simulink model "test_rig"  (Simulink 7.2)
settings: Solver=FixedStepDiscrete  StartTime=0.0  StopTime=55.0  FixedStep=0.5  RelTol=1e-3
libraries: simulink_need_slupdate x22, simulink x5, simulink_extras x1
settings Model: Creator=bjax  LastModifiedBy=bjax  ExtModeAutoUpdateStatusClock=off
settings DataIOCC: SignalLoggingName=sigsOut
settings OptimizationCC: InlineInvariantSignals=on  InitFltsAndDblsToZero=on
settings DebuggingCC: SaveWithParameterizedLinksMsg=none  SignalResolutionControl=TryResolveAllWithWarning  SolverPrmCheckMsg=none  MultiTaskDSMMsg=warning  MultiTaskCondExecSysMsg=none  StrictBusMsg=None
settings HardwareCC: TargetUnknown=on
settings RTWCC: IncludeERTFirstTime=on
settings GRTTargetCC: TargetFcnLib=ansi_tfl_tmw.mat  ModelReferenceCompliant=off  MatFileLogging=off

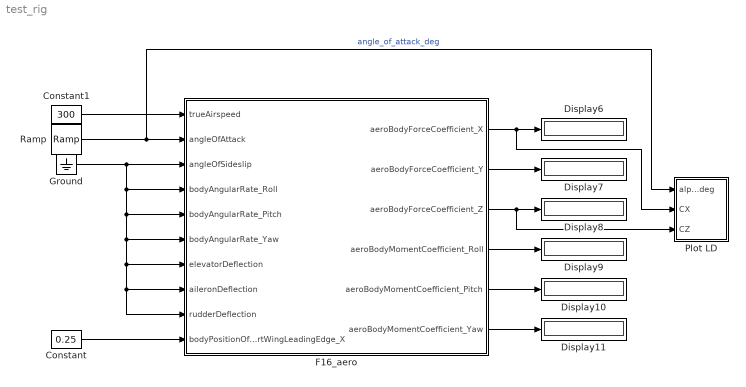
== system test_rig ==
  Constant : Constant  Value=0.25  OutDataType=sfix(16)  OutScaling=2^0
  Constant1 : Constant  Value=300  OutDataType=sfix(16)  OutScaling=2^0
  Display{6..11} (6 alike) : Display
  F16_aero : Subsystem
  Ground : Ground
  Plot LD : Subsystem
  Ramp : simulink/Sources/Ramp  SystemSampleTime=-1  slope=1  start=0  X0=-10
  wires:
  Ramp/1 -> Plot LD/1(alpha_deg), F16_aero/2(angleOfAttack)  "angle_of_attack_deg"
  F16_aero/2(aeroBodyForceCoefficient_Y) -> Display7/1
  F16_aero/3(aeroBodyForceCoefficient_Z) -> Display8/1, Plot LD/3(CZ)
  F16_aero/4(aeroBodyMomentCoefficient_Roll) -> Display9/1
  F16_aero/5(aeroBodyMomentCoefficient_Pitch) -> Display10/1
  F16_aero/6(aeroBodyMomentCoefficient_Yaw) -> Display11/1
  Constant/1 -> F16_aero/10(bodyPositionOfCgWrtWingLeadingEdge_X)
  Constant1/1 -> F16_aero/1(trueAirspeed)
  F16_aero/1(aeroBodyForceCoefficient_X) -> Display6/1, Plot LD/2(CX)
  Ground/1 -> F16_aero/8(aileronDeflection), F16_aero/9(rudderDeflection), F16_aero/7(elevatorDeflection), F16_aero/6(bodyAngularRate_Yaw), F16_aero/5(bodyAngularRate_Pitch), F16_aero/4(bodyAngularRate_Roll), F16_aero/3(angleOfSideslip)

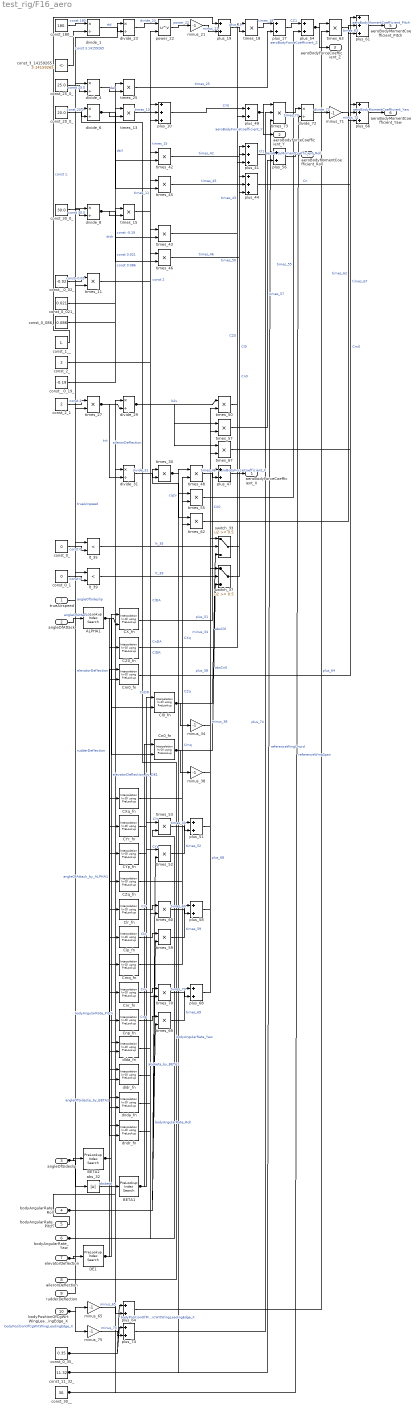
== system test_rig/F16_aero ==
  trueAirspeed : Inport
  angleOfAttack : Inport  Port=2
  angleOfSideslip : Inport  Port=3
  bodyAngularRate_Roll : Inport  Port=4
  bodyAngularRate_Pitch : Inport  Port=5
  bodyAngularRate_Yaw : Inport  Port=6
  elevatorDeflection : Inport  Port=7
  aileronDeflection : Inport  Port=8
  rudderDeflection : Inport  Port=9
  bodyPositionOfCgWrtWingLeadingEdge_X : Inport  Port=10
  ALPHA1 : simulink_need_slupdate/PreLookup Index Search  bpData=F16_aero_data.ALPHA1_pts  searchMode=Binary Search  cacheBpFlag=on  outputFlag=off  IndexDataType=uint32  extrapMode=Linear Extrapolation  rangeErrorMode=None
  BETA1 : simulink_need_slupdate/PreLookup Index Search  bpData=F16_aero_data.BETA1_pts  searchMode=Binary Search  cacheBpFlag=on  outputFlag=off  IndexDataType=uint32  extrapMode=Linear Extrapolation  rangeErrorMode=None
  BETA2 : simulink_need_slupdate/PreLookup Index Search  bpData=F16_aero_data.BETA2_pts  searchMode=Binary Search  cacheBpFlag=on  outputFlag=off  IndexDataType=uint32  extrapMode=Linear Extrapolation  rangeErrorMode=None
  CX_fn : simulink_need_slupdate/Interpolation (n-D) using PreLookup  numDimsPopupSelect=2  explicitNumDims=2  table=F16_aero_data.CX_table  interpMethod=Linear  extrapMethod=None - Clip  rangeErrorMode=None  NumSelectionDims=0
  CXq_fn : simulink_need_slupdate/Interpolation (n-D) using PreLookup  numDimsPopupSelect=1  explicitNumDims=1  table=F16_aero_data.CXq_table  interpMethod=Linear  extrapMethod=None - Clip  rangeErrorMode=None  NumSelectionDims=0
  CYp_fn : simulink_need_slupdate/Interpolation (n-D) using PreLookup  numDimsPopupSelect=1  explicitNumDims=1  table=F16_aero_data.CYp_table  interpMethod=Linear  extrapMethod=None - Clip  rangeErrorMode=None  NumSelectionDims=0
  CYr_fn : simulink_need_slupdate/Interpolation (n-D) using PreLookup  numDimsPopupSelect=1  explicitNumDims=1  table=F16_aero_data.CYr_table  interpMethod=Linear  extrapMethod=None - Clip  rangeErrorMode=None  NumSelectionDims=0
  CZ0_fn : simulink_need_slupdate/Interpolation (n-D) using PreLookup  numDimsPopupSelect=1  explicitNumDims=1  table=F16_aero_data.CZ0_table  interpMethod=Linear  extrapMethod=None - Clip  rangeErrorMode=None  NumSelectionDims=0
  CZq_fn : simulink_need_slupdate/Interpolation (n-D) using PreLookup  numDimsPopupSelect=1  explicitNumDims=1  table=F16_aero_data.CZq_table  interpMethod=Linear  extrapMethod=None - Clip  rangeErrorMode=None  NumSelectionDims=0
  Cl0_fn : simulink_need_slupdate/Interpolation (n-D) using PreLookup  numDimsPopupSelect=2  explicitNumDims=2  table=F16_aero_data.Cl0_table  interpMethod=Linear  extrapMethod=None - Clip  rangeErrorMode=None  NumSelectionDims=0
  Clp_fn : simulink_need_slupdate/Interpolation (n-D) using PreLookup  numDimsPopupSelect=1  explicitNumDims=1  table=F16_aero_data.Clp_table  interpMethod=Linear  extrapMethod=None - Clip  rangeErrorMode=None  NumSelectionDims=0
  Clr_fn : simulink_need_slupdate/Interpolation (n-D) using PreLookup  numDimsPopupSelect=1  explicitNumDims=1  table=F16_aero_data.Clr_table  interpMethod=Linear  extrapMethod=None - Clip  rangeErrorMode=None  NumSelectionDims=0
  Cm0_fn : simulink_need_slupdate/Interpolation (n-D) using PreLookup  numDimsPopupSelect=2  explicitNumDims=2  table=F16_aero_data.Cm0_table  interpMethod=Linear  extrapMethod=None - Clip  rangeErrorMode=None  NumSelectionDims=0
  Cmq_fn : simulink_need_slupdate/Interpolation (n-D) using PreLookup  numDimsPopupSelect=1  explicitNumDims=1  table=F16_aero_data.Cmq_table  interpMethod=Linear  extrapMethod=None - Clip  rangeErrorMode=None  NumSelectionDims=0
  Cn0_fn : simulink_need_slupdate/Interpolation (n-D) using PreLookup  numDimsPopupSelect=2  explicitNumDims=2  table=F16_aero_data.Cn0_table  interpMethod=Linear  extrapMethod=None - Clip  rangeErrorMode=None  NumSelectionDims=0
  Cnp_fn : simulink_need_slupdate/Interpolation (n-D) using PreLookup  numDimsPopupSelect=1  explicitNumDims=1  table=F16_aero_data.Cnp_table  interpMethod=Linear  extrapMethod=None - Clip  rangeErrorMode=None  NumSelectionDims=0
  Cnr_fn : simulink_need_slupdate/Interpolation (n-D) using PreLookup  numDimsPopupSelect=1  explicitNumDims=1  table=F16_aero_data.Cnr_table  interpMethod=Linear  extrapMethod=None - Clip  rangeErrorMode=None  NumSelectionDims=0
  DE1 : simulink_need_slupdate/PreLookup Index Search  bpData=F16_aero_data.DE1_pts  searchMode=Binary Search  cacheBpFlag=on  outputFlag=off  IndexDataType=uint32  extrapMode=Linear Extrapolation  rangeErrorMode=None
  abs_32 : Abs  SaturateOnIntegerOverflow=on
  const_0_ : Constant  Value=0
  const_0_021_ : Constant  Value=0.021
  const_0_086_ : Constant  Value=0.086
  const_0_1 : Constant  Value=0
  const_0_35_ : Constant  Value=0.35
  const_11_32_ : Constant  Value=11.32
  const_180__ : Constant  Value=180.
  const_1__ : Constant  Value=1.
  const_20_0_ : Constant  Value=20.0
  const_25_0_ : Constant  Value=25.0
  const_2_ : Constant  Value=2
  const_2_1 : Constant  Value=2
  const_30_0_ : Constant  Value=30.0
  const_30__ : Constant  Value=30.
  const_3_14159265_ : Constant  Value=3.14159265
  const__0_02_ : Constant  Value=-0.02
  const__0_19_ : Constant  Value=-0.19
  divide_{1,4,6,8,23,29,31,72} (8 alike) : Product  Inputs=*/  SaturateOnIntegerOverflow=on  RndMeth=Zero  InputSameDT=on  OutDataTypeStr=Inherit: Same as first input
  dlda_fn : simulink_need_slupdate/Interpolation (n-D) using PreLookup  numDimsPopupSelect=2  explicitNumDims=2  table=F16_aero_data.dlda_table  interpMethod=Linear  extrapMethod=None - Clip  rangeErrorMode=None  NumSelectionDims=0
  dldr_fn : simulink_need_slupdate/Interpolation (n-D) using PreLookup  numDimsPopupSelect=2  explicitNumDims=2  table=F16_aero_data.dldr_table  interpMethod=Linear  extrapMethod=None - Clip  rangeErrorMode=None  NumSelectionDims=0
  dnda_fn : simulink_need_slupdate/Interpolation (n-D) using PreLookup  numDimsPopupSelect=2  explicitNumDims=2  table=F16_aero_data.dnda_table  interpMethod=Linear  extrapMethod=None - Clip  rangeErrorMode=None  NumSelectionDims=0
  dndr_fn : simulink_need_slupdate/Interpolation (n-D) using PreLookup  numDimsPopupSelect=2  explicitNumDims=2  table=F16_aero_data.dndr_table  interpMethod=Linear  extrapMethod=None - Clip  rangeErrorMode=None  NumSelectionDims=0
  lt_35 : RelationalOperator  Operator=<  InputSameDT=on
  lt_39 : RelationalOperator  Operator=<  InputSameDT=on
  minus_{21,34,38,65,71,75} (6 alike) : Gain  Gain=-1  SaturateOnIntegerOverflow=on  OutDataTypeStr=Inherit: Same as input  ParamDataTypeStr=Inherit: Same as input
  plus_{10,41,44,61,66} (5 alike) : Sum  Inputs=+++  SaturateOnIntegerOverflow=on  InputSameDT=on  OutDataTypeStr=Inherit: Same as first input
  plus_{17,19,47,49,51,54,56,58,64,68,74} (11 alike) : Sum  SaturateOnIntegerOverflow=on  InputSameDT=on  OutDataTypeStr=Inherit: Same as first input
  power_22 : Math  Operator=pow  SaturateOnIntegerOverflow=on
  switch_33 : Switch  Threshold=0.5  SaturateOnIntegerOverflow=on  InputSameDT=on
  switch_37 : Switch  Threshold=0.5  SaturateOnIntegerOverflow=on  InputSameDT=on
  times_{11,13,15,18,25,27,30,42..43,45..46,48,50,52..53,55,57,59..60,62..63,67,69..70} (24 alike) : Product  SaturateOnIntegerOverflow=on  RndMeth=Zero  InputSameDT=on  OutDataTypeStr=Inherit: Same as first input
  times_73 : Product  Inputs=3  SaturateOnIntegerOverflow=on  RndMeth=Zero  InputSameDT=on  OutDataTypeStr=Inherit: Same as first input
  aeroBodyForceCoefficient_X : Outport
  aeroBodyForceCoefficient_Y : Outport  Port=2
  aeroBodyForceCoefficient_Z : Outport  Port=3
  aeroBodyMomentCoefficient_Roll : Outport  Port=4
  aeroBodyMomentCoefficient_Pitch : Outport  Port=5
  aeroBodyMomentCoefficient_Yaw : Outport  Port=6
  wires:
  BETA2/1 -> dndr_fn/1, dnda_fn/1, dldr_fn/1, dlda_fn/1  "angleOfSideslip_by_BETA2"
  BETA1/1 -> Cn0_fn/1, Cl0_fn/1  "absbeta_by_BETA1"
  ALPHA1/1 -> dndr_fn/2, dnda_fn/2, dldr_fn/2, dlda_fn/2, Cnp_fn/1, Cnr_fn/1, Cmq_fn/1, Clp_fn/1, Clr_fn/1, CZq_fn/1, CYp_fn/1, CYr_fn/1, CXq_fn/1, Cn0_fn/2, Cl0_fn/2, Cm0_fn/2, CZ0_fn/1, CX_fn/2  "angleOfAttack_by_ALPHA1"
  DE1/1 -> Cm0_fn/1, CX_fn/1  "elevatorDeflection_by_DE1"
  minus_75/1 -> plus_74/2  "minus_75"
  plus_74/1 -> times_73/2  "plus_74"
  times_73/1 -> divide_72/1  "times_73"
  divide_72/1 -> minus_71/1  "divide_72"
  minus_71/1 -> plus_66/3  "minus_71"
  times_70/1 -> plus_68/2  "times_70"
  times_69/1 -> plus_68/1  "times_69"
  plus_68/1 -> times_67/2  "plus_68"
  times_67/1 -> plus_66/2  "times_67"
  plus_66/1 -> aeroBodyMomentCoefficient_Yaw/1  "aeroBodyMomentCoefficient_Yaw"
  minus_65/1 -> plus_64/2  "minus_65"
  plus_64/1 -> times_63/2  "plus_64"
  times_63/1 -> plus_61/3  "times_63"
  times_62/1 -> plus_61/2  "times_62"
  plus_61/1 -> aeroBodyMomentCoefficient_Pitch/1  "aeroBodyMomentCoefficient_Pitch"
  times_60/1 -> plus_58/2  "times_60"
  times_59/1 -> plus_58/1  "times_59"
  plus_58/1 -> times_57/2  "plus_58"
  times_57/1 -> plus_56/2  "times_57"
  plus_56/1 -> aeroBodyMomentCoefficient_Roll/1  "aeroBodyMomentCoefficient_Roll"
  times_55/1 -> plus_54/2  "times_55"
  plus_54/1 -> aeroBodyForceCoefficient_Z/1, times_63/1  "aeroBodyForceCoefficient_Z"
  times_53/1 -> plus_51/2  "times_53"
  times_52/1 -> plus_51/1  "times_52"
  plus_51/1 -> times_50/2  "plus_51"
  times_50/1 -> plus_49/2  "times_50"
  plus_49/1 -> aeroBodyForceCoefficient_Y/1, times_73/1  "aeroBodyForceCoefficient_Y"
  times_48/1 -> plus_47/2  "times_48"
  plus_47/1 -> aeroBodyForceCoefficient_X/1  "aeroBodyForceCoefficient_X"
  times_46/1 -> plus_44/3  "times_46"
  times_45/1 -> plus_44/2  "times_45"
  plus_44/1 -> plus_66/1  "Cn"
  times_43/1 -> plus_41/3  "times_43"
  times_42/1 -> plus_41/2  "times_42"
  plus_41/1 -> plus_56/1  "Cl1"
  dndr_fn/1 -> times_46/1  "CnDR"
  dnda_fn/1 -> times_45/1  "CnDA"
  dldr_fn/1 -> times_43/1  "ClDR"
  dlda_fn/1 -> times_42/1  "ClDA"
  Cnp_fn/1 -> times_69/1  "Cnp"
  Cnr_fn/1 -> times_70/1  "Cnr"
  Cmq_fn/1 -> times_62/2  "Cmq"
  Clp_fn/1 -> times_59/1  "Clp"
  Clr_fn/1 -> times_60/1  "Clr"
  CZq_fn/1 -> times_55/2  "CZq"
  CYp_fn/1 -> times_52/1  "CYp"
  CYr_fn/1 -> times_53/1  "CYr"
  CXq_fn/1 -> times_48/2  "CXq"
  const_0_1/1 -> lt_39/2  "const 0"
  lt_39/1 -> switch_37/2  "lt_39"
  minus_38/1 -> switch_37/1  "minus_38"
  switch_37/1 -> plus_44/1  "Cn0"
  Cm0_fn/1 -> plus_61/1  "Cm0"
  const_0_/1 -> lt_35/2  "const 0"
  lt_35/1 -> switch_33/2  "lt_35"
  minus_34/1 -> switch_33/1  "minus_34"
  switch_33/1 -> plus_41/1  "Cl0"
  Cn0_fn/1 -> minus_38/1, switch_37/3  "absCn0"
  Cl0_fn/1 -> minus_34/1, switch_33/3  "absCl0"
  abs_32/1 -> BETA1/1  "absbeta"
  divide_31/1 -> times_30/2  "divide_31"
  times_30/1 -> times_62/1, times_55/1, times_48/1  "cq2v"
  divide_29/1 -> times_67/1, times_57/1, times_50/1  "b2v"
  const_2_1/1 -> times_27/1  "const 2"
  times_27/1 -> divide_31/2, divide_29/2  "tvt"
  const__0_19_/1 -> times_25/1  "const -0.19"
  times_25/1 -> plus_17/2  "times_25"
  const_2_/1 -> power_22/2  "const 2"
  divide_23/1 -> power_22/1  "divide_23"
  power_22/1 -> minus_21/1  "power_22"
  minus_21/1 -> plus_19/2  "minus_21"
  const_1__/1 -> plus_19/1  "const 1."
  plus_19/1 -> times_18/2  "plus_19"
  times_18/1 -> plus_17/1  "times_18"
  plus_17/1 -> plus_54/1  "CZ1"
  CZ0_fn/1 -> times_18/1  "CZ0"
  const_0_086_/1 -> times_15/1  "const 0.086"
  times_15/1 -> plus_10/3  "times_15"
  const_0_021_/1 -> times_13/1  "const 0.021"
  times_13/1 -> plus_10/2  "times_13"
  const__0_02_/1 -> times_11/1  "const -0.02"
  times_11/1 -> plus_10/1  "times_11"
  plus_10/1 -> plus_49/1  "CY0"
  CX_fn/1 -> plus_47/1  "CX0"
  const_30_0_/1 -> divide_8/2  "const 30.0"
  divide_8/1 -> times_46/2, times_43/2, times_15/2  "drdr"
  const_20_0_/1 -> divide_6/2  "const 20.0"
  divide_6/1 -> times_45/2, times_42/2, times_13/2  "dail"
  const_25_0_/1 -> divide_4/2  "const 25.0"
  divide_4/1 -> times_25/2  "del"
  const_30__/1 -> divide_72/2, divide_29/1  "referenceWingSpan"
  const_11_32_/1 -> times_73/3, times_30/1  "referenceWingChord"
  const_0_35_/1 -> plus_74/1, plus_64/1  "bodyPositionOfMrcWrtWingLeadingEdge_X"
  const_3_14159265_/1 -> divide_1/2  "const 3.14159265"
  const_180__/1 -> divide_1/1  "const 180."
  divide_1/1 -> divide_23/2  "rtd"
  bodyPositionOfCgWrtWingLeadingEdge_X/1 -> minus_75/1, minus_65/1  "bodyPositionOfCgWrtWingLeadingEdge_X"
  rudderDeflection/1 -> divide_8/1  "rudderDeflection"
  aileronDeflection/1 -> divide_6/1  "aileronDeflection"
  elevatorDeflection/1 -> divide_4/1, DE1/1  "elevatorDeflection"
  bodyAngularRate_Yaw/1 -> times_70/2, times_60/2, times_53/2  "bodyAngularRate_Yaw"
  bodyAngularRate_Pitch/1 -> divide_31/1  "bodyAngularRate_Pitch"
  bodyAngularRate_Roll/1 -> times_69/2, times_59/2, times_52/2  "bodyAngularRate_Roll"
  angleOfSideslip/1 -> lt_39/1, lt_35/1, abs_32/1, divide_23/1, times_11/2, BETA2/1  "angleOfSideslip"
  angleOfAttack/1 -> ALPHA1/1  "angleOfAttack"
  trueAirspeed/1 -> times_27/2  "trueAirspeed"

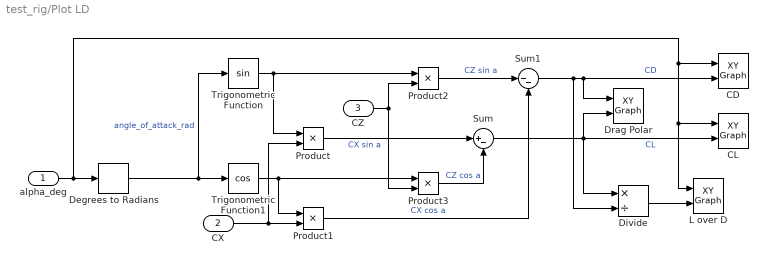
== system test_rig/Plot LD ==
  alpha_deg : Inport  OutDataType=sfix(16)  OutScaling=2^0
  CX : Inport  Port=2  OutDataType=sfix(16)  OutScaling=2^0
  CZ : Inport  Port=3  OutDataType=sfix(16)  OutScaling=2^0
  CD : simulink/Sinks/XY Graph  SystemSampleTime=-1  xmin=-10  xmax=45  ymin=0  ymax=2  st=-1
  CL : simulink/Sinks/XY Graph  SystemSampleTime=-1  xmin=-10  xmax=45  ymin=-1  ymax=2  st=-1
  Degrees to Radians : simulink_extras/Transformations/Degrees to Radians  SystemSampleTime=-1
  Divide : Product  Inputs=*/  OutDataType=sfix(16)  OutScaling=2^-10
  Drag Polar : simulink/Sinks/XY Graph  SystemSampleTime=-1  xmin=0  xmax=1.5  ymin=-1  ymax=2  st=-1
  L over D : simulink/Sinks/XY Graph  SystemSampleTime=-1  xmin=-10  xmax=45  ymin=0  ymax=15  st=-1
  Product{,1..3} (4 alike) : Product  OutDataType=sfix(16)  OutScaling=2^0  SaturateOnIntegerOverflow=on  OutDataTypeStr=Inherit: Same as first input
  Sum : Sum  Inputs=|+-  OutDataType=sfix(16)  OutScaling=2^0  SaturateOnIntegerOverflow=on
  Sum1 : Sum  Inputs=|--  OutDataType=sfix(16)  OutScaling=2^0  SaturateOnIntegerOverflow=on
  Trigonometric Function : Trigonometry
  Trigonometric Function1 : Trigonometry  Operator=cos
  wires:
  Degrees to Radians/1 -> Trigonometric Function1/1, Trigonometric Function/1  "angle_of_attack_rad"
  Trigonometric Function/1 -> Product/1, Product2/1
  Trigonometric Function1/1 -> Product1/1, Product3/1
  Product/1 -> Sum/1  "CX sin a"
  Product3/1 -> Sum/2  "CZ cos a"
  Product2/1 -> Sum1/1  "CZ sin a"
  Product1/1 -> Sum1/2  "CX cos a"
  alpha_deg/1 -> Degrees to Radians/1, CD/1, CL/1, L over D/1
  CZ/1 -> Product2/2, Product3/2
  CX/1 -> Product/2, Product1/2
  Sum1/1 -> CD/2, Drag Polar/1, Divide/2  "CD"
  Sum/1 -> CL/2, Drag Polar/2, Divide/1  "CL"
  Divide/1 -> L over D/2
